simulink model "Car_Blinker"  (R2022b)
settings: Solver=FixedStepAuto  StartTime=0.0  StopTime=inf  RelTol=1e-3
libraries: arduinolib x5, simulink x3
settings Model: ExtModeTrigDuration=2  Creator=MAAM  LastModifiedBy=MAAM
settings OptimizationCC: EnhancedBackFolding=on  PassReuseOutputArgsAs=Individual arguments  ZeroExternalMemoryAtStartup=off  ZeroInternalMemoryAtStartup=off  MaxStackSize=64  OptimizeBlockOrder=speed  DifferentSizesBufferReuse=on  OptimizationCustomize=off  EfficientTunableParamExpr=on
settings DebuggingCC: ParameterTunabilityLossMsg=error
settings HardwareCC: ProdBitPerInt=16  ProdBitPerPointer=16  ProdBitPerSizeT=16  ProdBitPerPtrDiffT=16  ProdLargestAtomicFloat=None  ProdWordSize=8  ProdHWDeviceType=Atmel->AVR
settings SFSimCC: MATLABDynamicMemAlloc=off
settings RTWCC: Description=Embedded Coder  SystemTargetFile=ert.tlc  HardwareBoard=Arduino Mega 2560  TemplateMakefile=ert_default_tmf  Toolchain=Arduino AVR  BuildConfiguration=Faster Runs
settings CodeAppCC: ForceParamTrailComments=on  IgnoreCustomStorageClasses=off  OperatorAnnotations=on  SimulinkDataObjDesc=on  SFDataObjDesc=on  InsertBlockDesc=on
settings ERTTargetCC: SupportContinuousTime=on  SupportVariableSizeSignals=on  ExtMode=on  ExtModeTransport=3  ExtModeStaticAlloc=on  ExtModeAutomaticAllocSize=off  ExtModeStaticAllocSize=2048  ExtModeMexFile=ext_xcp  ExtModeMexArgs=0 5 921600  ExtModeIntrfLevel=Level2 - Open

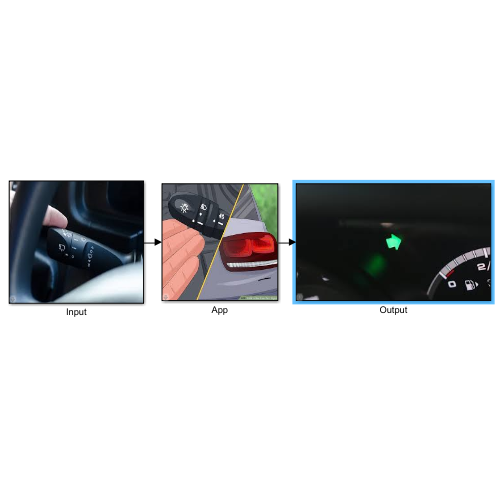
[thumbnail: Simulink's stored preview of the top-level diagram]
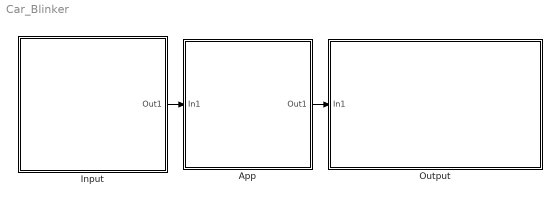
== system Car_Blinker ==
  App : Subsystem  mask{D_time=10, B_freq=0.5}
      mask prompts: D_time "Button Debouncing delay time (steps)"; B_freq "Light Blinking Freq (Hz)"
      mask Display: image("blinker_system.jpg");
  Input : Subsystem  mask{l_pin=3, r_pin=2, w_pin=4}
      mask prompts: l_pin "Left input pin (<<)"; r_pin "Right input pin (>>)"; w_pin "Waiting input pin (<!>)"
      mask Display: image("blinker_input.jpg")
  Output : Subsystem  mask{l_pin=10, r_pin=9}
      mask prompts: l_pin "Left Light output (<<)"; r_pin "Right Light output (>>)"
      mask Display: image("blinker_output.jpg");
  wires:
  Input/1(Out1) -> App/1(In1)
  App/1(Out1) -> Output/1(In1)

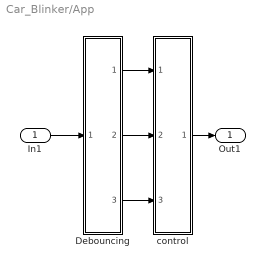
== system Car_Blinker/App ==
  In1 : Inport
  Debouncing : Subsystem
  control : Subsystem
  Out1 : Outport
  wires:
  Debouncing/3(Out3) -> control/3(In3)
  Debouncing/1(Out1) -> control/1(In1)
  control/1(OutBus) -> Out1/1
  Debouncing/2(Out2) -> control/2(In2)
  In1/1 -> Debouncing/1(InBus)

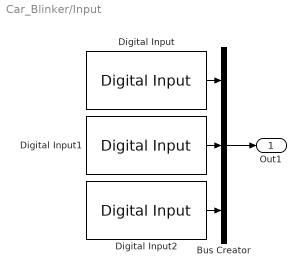
== system Car_Blinker/Input ==
  Bus Creator : BusCreator  Inputs=3
  Digital Input : arduinolib/Digital Input  pinNumber=w_pin  mode=Default  Direction=input  SampleTime=0.1  blockPlatform=arduino
  Digital Input1 : arduinolib/Digital Input  pinNumber=l_pin  mode=Default  Direction=input  SampleTime=0.1  blockPlatform=arduino
  Digital Input2 : arduinolib/Digital Input  pinNumber=r_pin  mode=Default  Direction=input  SampleTime=0.1  blockPlatform=arduino
  Out1 : Outport
  wires:
  Digital Input/1 -> Bus Creator/1
  Digital Input2/1 -> Bus Creator/3
  Digital Input1/1 -> Bus Creator/2
  Bus Creator/1 -> Out1/1

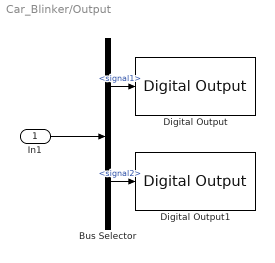
== system Car_Blinker/Output ==
  In1 : Inport
  Bus Selector : BusSelector  OutputSignals=signal1,signal2
  Digital Output : arduinolib/Digital Output  pinNumber=l_pin  Direction=output  blockPlatform=arduino
  Digital Output1 : arduinolib/Digital Output  pinNumber=r_pin  Direction=output  blockPlatform=arduino
  wires:
  Bus Selector/1 -> Digital Output/1  "<signal1>"
  Bus Selector/2 -> Digital Output1/1  "<signal2>"
  In1/1 -> Bus Selector/1

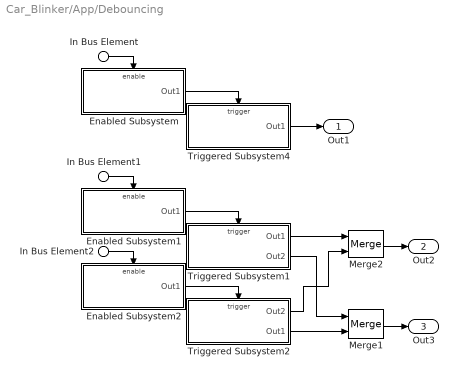
== system Car_Blinker/App/Debouncing ==
  In Bus Element : Inport  PortName=InBus  Element=signal1
  In Bus Element1 : Inport  PortName=InBus  Element=signal2
  In Bus Element2 : Inport  PortName=InBus  Element=signal3
  Enabled Subsystem : Subsystem  TreatAsAtomicUnit=on
  Enabled Subsystem1 : Subsystem  TreatAsAtomicUnit=on
  Enabled Subsystem2 : Subsystem  TreatAsAtomicUnit=on
  Merge1 : Merge
  Merge2 : Merge
  Triggered Subsystem1 : Subsystem  TreatAsAtomicUnit=on
  Triggered Subsystem2 : Subsystem  TreatAsAtomicUnit=on
  Triggered Subsystem4 : Subsystem  TreatAsAtomicUnit=on
  Out1 : Outport
  Out2 : Outport  Port=2
  Out3 : Outport  Port=3
  wires:
  Triggered Subsystem4/1(Out1) -> Out1/1
  Enabled Subsystem/1(Out1) -> Triggered Subsystem4/Trigger
  In Bus Element/1 -> Enabled Subsystem/Enable
  In Bus Element1/1 -> Enabled Subsystem1/Enable
  In Bus Element2/1 -> Enabled Subsystem2/Enable
  Merge1/1 -> Out3/1
  Merge2/1 -> Out2/1
  Enabled Subsystem1/1(Out1) -> Triggered Subsystem1/Trigger
  Enabled Subsystem2/1(Out1) -> Triggered Subsystem2/Trigger
  Triggered Subsystem1/1(Out1) -> Merge2/1
  Triggered Subsystem2/1(Out2) -> Merge2/2
  Triggered Subsystem2/2(Out1) -> Merge1/2
  Triggered Subsystem1/2(Out2) -> Merge1/1

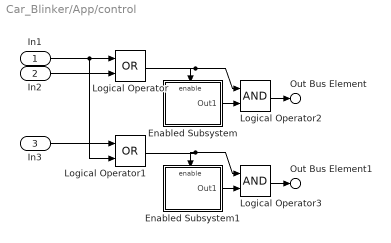
== system Car_Blinker/App/control ==
  In1 : Inport
  In2 : Inport  Port=2
  In3 : Inport  Port=3
  Enabled Subsystem : Subsystem  TreatAsAtomicUnit=on
  Enabled Subsystem1 : Subsystem  TreatAsAtomicUnit=on
  Logical Operator : Logic  Operator=OR  AllPortsSameDT=off  OutDataTypeStr=boolean
  Logical Operator1 : Logic  Operator=OR  AllPortsSameDT=off  OutDataTypeStr=boolean
  Logical Operator2 : Logic  AllPortsSameDT=off  OutDataTypeStr=boolean
  Logical Operator3 : Logic  AllPortsSameDT=off  OutDataTypeStr=boolean
  Out Bus Element : Outport  PortName=OutBus  Element=signal1
  Out Bus Element1 : Outport  PortName=OutBus  Element=signal2
  wires:
  In1/1 -> Logical Operator1/2, Logical Operator/1
  Logical Operator/1 -> Logical Operator2/1, Enabled Subsystem/Enable
  In2/1 -> Logical Operator/2
  In3/1 -> Logical Operator1/1
  Logical Operator1/1 -> Logical Operator3/1, Enabled Subsystem1/Enable
  Enabled Subsystem/1(Out1) -> Logical Operator2/2
  Enabled Subsystem1/1(Out1) -> Logical Operator3/2
  Logical Operator2/1 -> Out Bus Element/1
  Logical Operator3/1 -> Out Bus Element1/1

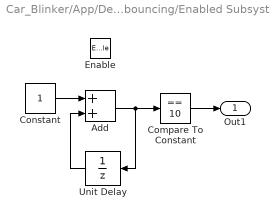
== system Car_Blinker/App/Debouncing/Enabled Subsystem ==
  Enable : EnablePort  StatesWhenEnabling=reset
  Add : Sum
  Compare To Constant : simulink/Logic and Bit Operations/Compare To Constant  relop===  const=10  OutDataTypeStr=boolean
  Constant : Constant
  Unit Delay : UnitDelay  SampleTime=0.1  HasFrameUpgradeWarning=on
  Out1 : Outport
  wires:
  Constant/1 -> Add/1
  Add/1 -> Unit Delay/1, Compare To Constant/1
  Unit Delay/1 -> Add/2
  Compare To Constant/1 -> Out1/1

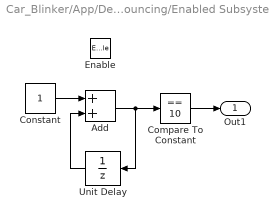
== system Car_Blinker/App/Debouncing/Enabled Subsystem1 ==
  Enable : EnablePort  StatesWhenEnabling=reset
  Add : Sum
  Compare To Constant : simulink/Logic and Bit Operations/Compare To Constant  relop===  const=10  OutDataTypeStr=boolean
  Constant : Constant
  Unit Delay : UnitDelay  SampleTime=0.1  HasFrameUpgradeWarning=on
  Out1 : Outport
  wires:
  Compare To Constant/1 -> Out1/1
  Unit Delay/1 -> Add/2
  Add/1 -> Compare To Constant/1, Unit Delay/1
  Constant/1 -> Add/1

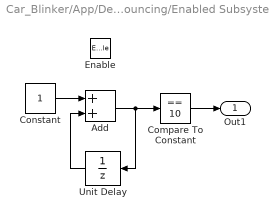
== system Car_Blinker/App/Debouncing/Enabled Subsystem2 ==
  Enable : EnablePort  StatesWhenEnabling=reset
  Add : Sum
  Compare To Constant : simulink/Logic and Bit Operations/Compare To Constant  relop===  const=10  OutDataTypeStr=boolean
  Constant : Constant
  Unit Delay : UnitDelay  SampleTime=0.1  HasFrameUpgradeWarning=on
  Out1 : Outport
  wires:
  Constant/1 -> Add/1
  Add/1 -> Unit Delay/1, Compare To Constant/1
  Unit Delay/1 -> Add/2
  Compare To Constant/1 -> Out1/1

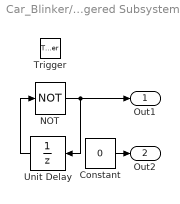
== system Car_Blinker/App/Debouncing/Triggered Subsystem1 ==
  Trigger : TriggerPort  VariantControl=(inherit)
  Constant : Constant  Value=0  OutDataTypeStr=boolean
  NOT : Logic  Operator=NOT  IconShape=distinctive  AllPortsSameDT=off  OutDataTypeStr=boolean
  Unit Delay : UnitDelay  SampleTime=-1  HasFrameUpgradeWarning=on
  Out1 : Outport
  Out2 : Outport  Port=2
  wires:
  Unit Delay/1 -> NOT/1
  NOT/1 -> Unit Delay/1, Out1/1
  Constant/1 -> Out2/1

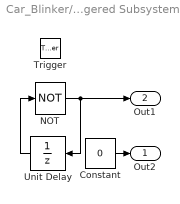
== system Car_Blinker/App/Debouncing/Triggered Subsystem2 ==
  Trigger : TriggerPort  VariantControl=(inherit)
  Constant : Constant  Value=0  OutDataTypeStr=boolean
  NOT : Logic  Operator=NOT  IconShape=distinctive  AllPortsSameDT=off  OutDataTypeStr=boolean
  Unit Delay : UnitDelay  SampleTime=-1  HasFrameUpgradeWarning=on
  Out2 : Outport
  Out1 : Outport  Port=2
  wires:
  Constant/1 -> Out2/1
  NOT/1 -> Out1/1, Unit Delay/1
  Unit Delay/1 -> NOT/1

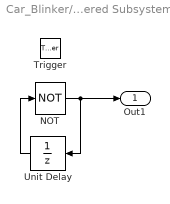
== system Car_Blinker/App/Debouncing/Triggered Subsystem4 ==
  Trigger : TriggerPort  VariantControl=(inherit)
  NOT : Logic  Operator=NOT  IconShape=distinctive  AllPortsSameDT=off  OutDataTypeStr=boolean
  Unit Delay : UnitDelay  SampleTime=-1  HasFrameUpgradeWarning=on
  Out1 : Outport
  wires:
  NOT/1 -> Out1/1, Unit Delay/1
  Unit Delay/1 -> NOT/1

== system Car_Blinker/App/control/Enabled Subsystem ==
  Enable : EnablePort
  Pulse Generator : DiscretePulseGenerator  PulseType=Time based  Period=1  PulseWidth=50
  Out1 : Outport
  wires:
  Pulse Generator/1 -> Out1/1

== system Car_Blinker/App/control/Enabled Subsystem1 ==
  Enable : EnablePort
  Pulse Generator : DiscretePulseGenerator  PulseType=Time based  Period=1  PulseWidth=50
  Out1 : Outport
  wires:
  Pulse Generator/1 -> Out1/1
